simulink model "pfd2"  (R2024b)
settings: Solver=VariableStepAuto  StartTime=0.0  StopTime=10.0  RelTol=1e-3
settings Model: Creator=marti  LastModifiedBy=marti

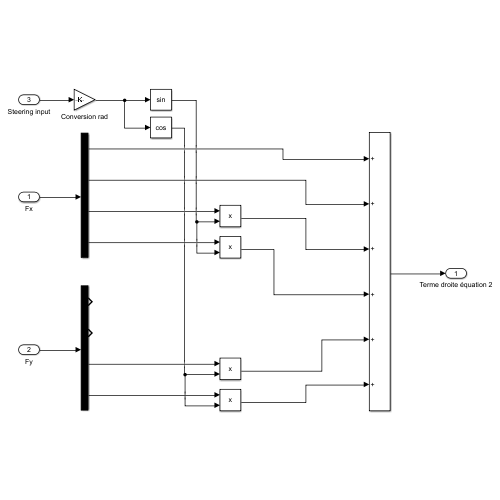
[thumbnail: Simulink's stored preview of the top-level diagram]
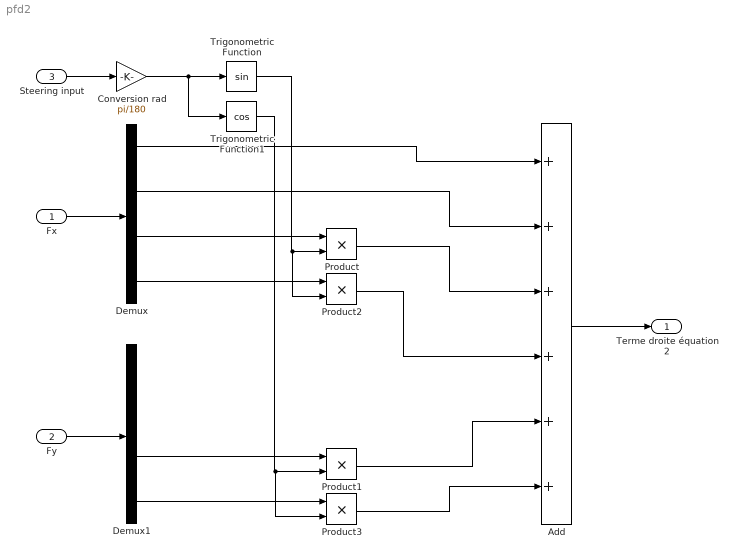
== system pfd2 ==
  Fx : Inport
  Fy : Inport  Port=2
  Steering input : Inport  Port=3
  Add : Sum  Inputs=++++++
  Conversion rad : Gain  Gain=pi/180
  Demux : Demux
  Demux1 : Demux
  Product{,1..3} (4 alike) : Product
  Trigonometric Function : Trigonometry
  Trigonometric Function1 : Trigonometry  Operator=cos
  Terme droite équation 2 : Outport
  wires:
  Steering input/1 -> Conversion rad/1
  Demux/3 -> Product/1
  Demux/1 -> Add/1
  Product2/1 -> Add/4
  Trigonometric Function1/1 -> Product3/2, Product1/2
  Demux/4 -> Product2/1
  Conversion rad/1 -> Trigonometric Function1/1, Trigonometric Function/1
  Fy/1 -> Demux1/1
  Fx/1 -> Demux/1
  Trigonometric Function/1 -> Product2/2, Product/2
  Product3/1 -> Add/6
  Product1/1 -> Add/5
  Demux1/3 -> Product1/1
  Demux1/4 -> Product3/1
  Product/1 -> Add/3
  Demux/2 -> Add/2
  Add/1 -> Terme droite équation 2/1
